simulink model "validation_simulations"  (R2019b)
settings: Solver=FixedStepAuto  StartTime=0.0  StopTime=stopTime  FixedStep=0.002  RelTol=1e-3
values from neighbouring files (symbols this model uses):
  Ao = A-L*C    [StabilizationControl.m]
  Bo = [B,L]    [StabilizationControl.m]
  Co = eye(4)    [StabilizationControl.m]
  Klqi_int = Klqi(5)    [StabilizationControl.m]
  Klqi_state = Klqi(1:4)    [StabilizationControl.m]
  Kpp_int = Kpp_i(5)    [StabilizationControl.m]
  Kpp_state = Kpp_i(1:4)    [StabilizationControl.m]
undefined symbols (not defined in the file or in its folder): ampl, ContrMethod, frequency, kalmf, Parameters
settings Model: Creator=Samsung  LastModifiedBy=Galbanyno

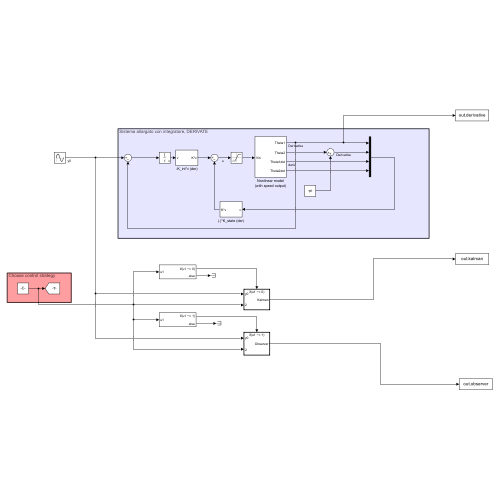
[thumbnail: Simulink's stored preview of the top-level diagram]
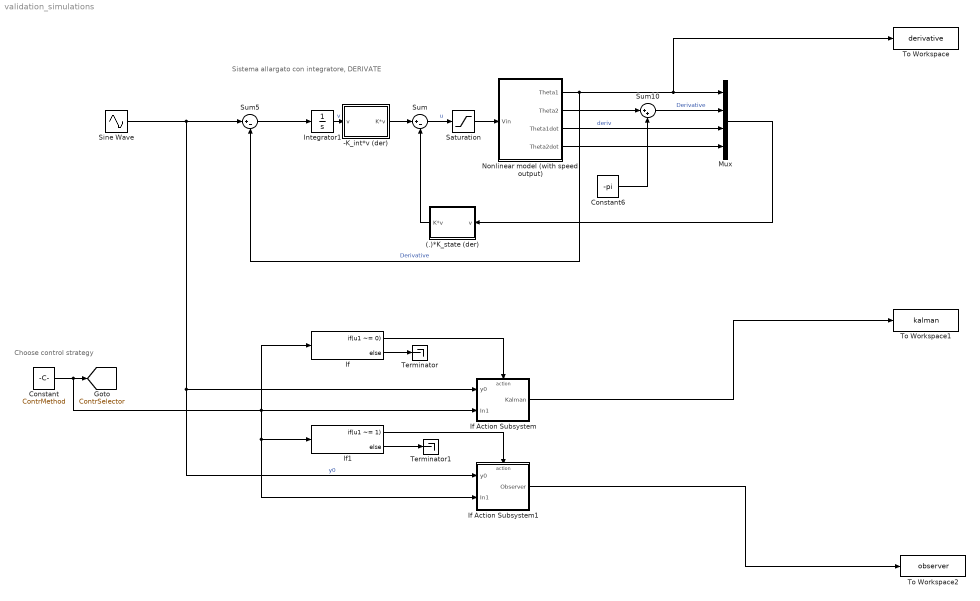
== system validation_simulations ==
  note: Choose control strategy
  note: Sistema allargato con integratore, DERIVATE
  "(.)*K_state (der) " : Subsystem
  -K_int*v (der) : Subsystem
  Constant : Constant  Value=ContrMethod
  Constant6 : Constant  Value=-pi
  If : If  IfExpression=u1 ~= 0
  If Action Subsystem : Subsystem  TreatAsAtomicUnit=on
  If Action Subsystem1 : Subsystem  TreatAsAtomicUnit=on
  If1 : If  IfExpression=u1 ~= 1
  Integrator1 : Integrator
  Mux : Mux
  Nonlinear model (with speed output) : Subsystem
  Saturation : Saturate  UpperLimit=10  LowerLimit=-10
  Sine Wave : Sin  Amplitude=ampl  Frequency=frequency  SampleTime=0
  Sum : Sum  Inputs=|+-
  Sum10 : Sum  Inputs=|++
  Sum5 : Sum  Inputs=|+-
  Terminator : Terminator
  Terminator1 : Terminator
  To Workspace : ToWorkspace  VariableName=derivative  SampleTime=-1
  To Workspace1 : ToWorkspace  VariableName=kalman  SampleTime=-1
  To Workspace2 : ToWorkspace  VariableName=observer  SampleTime=-1
  tag scope: ContrSelector=global
  wires:
  Nonlinear model (with speed output)/2(Theta2) -> Sum10/1
  "(.)*K_state (der) "/1(K*v) -> Sum/2
  Sum/1 -> Saturation/1  "u"
  Constant6/1 -> Sum10/2
  Integrator1/1 -> -K_int*v (der)/1(v)  "v"
  -K_int*v (der)/1(K*v) -> Sum/1
  Saturation/1 -> Nonlinear model (with speed output)/1(Vin)
  Sine Wave/1 -> If Action Subsystem1/1(y0), If Action Subsystem/1(y0), Sum5/1  "y0"
  Constant/1 -> If Action Subsystem/2(In1), If Action Subsystem1/2(In1), If1/1, If/1, [ContrSelector]
  Nonlinear model (with speed output)/1(Theta1) -> To Workspace/1, Mux/1, Sum5/2  "Derivative"
  Sum10/1 -> Mux/2  "Derivative"
  Nonlinear model (with speed output)/3(Theta1dot) -> Mux/3  "deriv"
  Nonlinear model (with speed output)/4(Theta2dot) -> Mux/4
  Mux/1 -> "(.)*K_state (der) "/1(v)
  Sum5/1 -> Integrator1/1
  If Action Subsystem/1(Kalman) -> To Workspace1/1
  If/1 -> If Action Subsystem/Action
  If Action Subsystem1/1(Observer) -> To Workspace2/1
  If/2 -> Terminator/1
  If1/2 -> Terminator1/1
  If1/1 -> If Action Subsystem1/Action

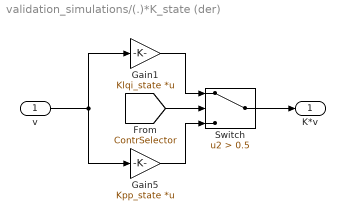
== system validation_simulations/(.)*K_state (der)  ==
  v : Inport
  Gain1 : Gain  Gain=Klqi_state  Multiplication=Matrix(K*u)
  Gain5 : Gain  Gain=Kpp_state  Multiplication=Matrix(K*u)
  Switch : Switch  Criteria=u2 > Threshold  Threshold=0.5
  K*v : Outport
  wires:
  Switch/1 -> K*v/1
  Gain5/1 -> Switch/3
  Gain1/1 -> Switch/1
  v/1 -> Gain5/1, Gain1/1
  [ContrSelector] -> Switch/2

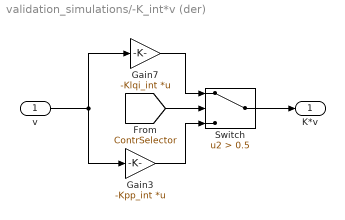
== system validation_simulations/-K_int*v (der) ==
  v : Inport
  Gain3 : Gain  Gain=-Kpp_int  Multiplication=Matrix(K*u)
  Gain7 : Gain  Gain=-Klqi_int  Multiplication=Matrix(K*u)
  Switch : Switch  Criteria=u2 > Threshold  Threshold=0.5
  K*v : Outport
  wires:
  Switch/1 -> K*v/1
  Gain3/1 -> Switch/3
  Gain7/1 -> Switch/1
  v/1 -> Gain3/1, Gain7/1
  [ContrSelector] -> Switch/2

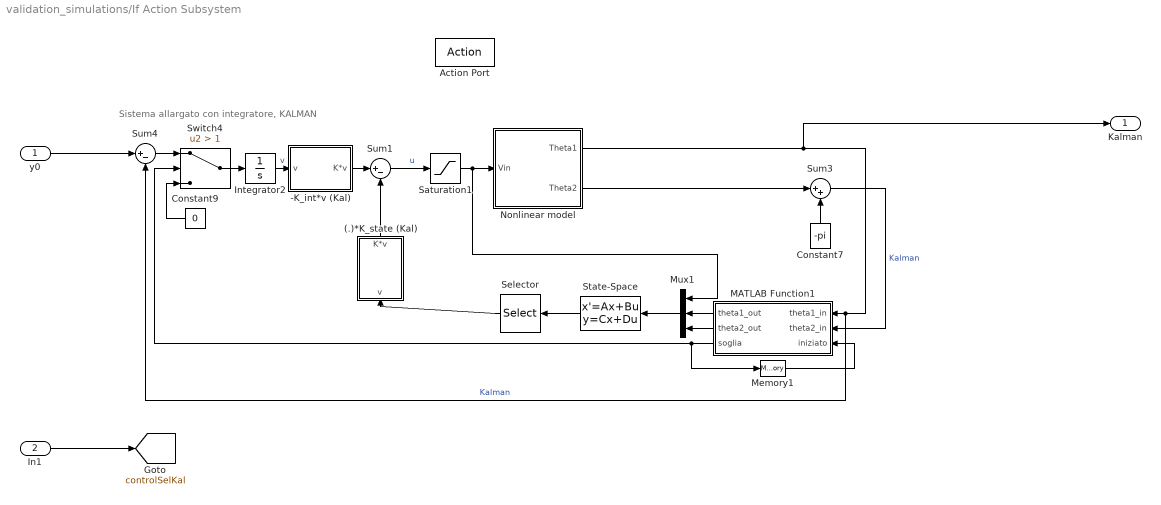
== system validation_simulations/If Action Subsystem ==
  note: Sistema allargato con integratore, KALMAN
  y0 : Inport
  In1 : Inport  Port=2
  Action Port : ActionPort  ActionPortLabel=if(u1 ~= 0)
  (.)*K_state (Kal) : Subsystem
  -K_int*v (Kal) : Subsystem
  Constant7 : Constant  Value=-pi
  Constant9 : Constant  Value=0
  Integrator2 : Integrator
  MATLAB Function1 : MATLAB Function  TreatAsAtomicUnit=on
  Memory1 : Memory  InitialCondition=false
  Mux1 : Mux  Inputs=3
  Nonlinear model : Subsystem
  Saturation1 : Saturate  UpperLimit=10  LowerLimit=-10
  Selector : Selector  InputPortWidth=6  IndexOptions=Index vector (dialog)  Indices=[3,4,5,6]  OutputSizes=1
  State-Space : StateSpace  A=kalmf.A  B=kalmf.B  C=kalmf.C  D=kalmf.D  InitialCondition=[0,0,0,0]
  Sum1 : Sum  Inputs=|+-
  Sum3 : Sum  Inputs=|++
  Sum4 : Sum  Inputs=|+-
  Switch4 : Switch  Criteria=u2 > Threshold  Threshold=1
  Kalman : Outport
  tag scope: controlSelKal=global
  wires:
  Selector/1 -> (.)*K_state (Kal)/1(v)
  Nonlinear model/2(Theta2) -> Sum3/1
  MATLAB Function1/2(theta2_out) -> Mux1/3
  (.)*K_state (Kal)/1(K*v) -> Sum1/2
  Integrator2/1 -> -K_int*v (Kal)/1(v)  "v"
  Sum3/1 -> MATLAB Function1/2(theta2_in)  "Kalman"
  Sum4/1 -> Switch4/1
  -K_int*v (Kal)/1(K*v) -> Sum1/1
  Switch4/1 -> Integrator2/1
  Constant9/1 -> Switch4/3
  Memory1/1 -> MATLAB Function1/3(iniziato)
  State-Space/1 -> Selector/1
  y0/1 -> Sum4/1
  Sum1/1 -> Saturation1/1  "u"
  MATLAB Function1/1(theta1_out) -> Mux1/2
  In1/1 -> [controlSelKal]
  Saturation1/1 -> Mux1/1, Nonlinear model/1(Vin)
  Nonlinear model/1(Theta1) -> Kalman/1, MATLAB Function1/1(theta1_in), Sum4/2  "Kalman"
  MATLAB Function1/3(soglia) -> Memory1/1, Switch4/2
  Mux1/1 -> State-Space/1
  Constant7/1 -> Sum3/2

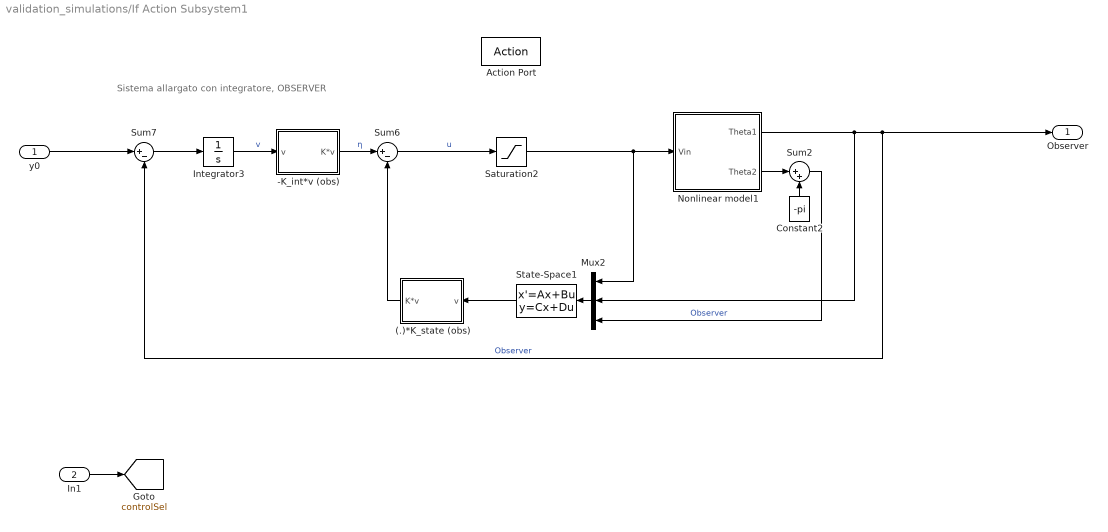
== system validation_simulations/If Action Subsystem1 ==
  note: Sistema allargato con integratore, OBSERVER
  y0 : Inport
  In1 : Inport  Port=2
  Action Port : ActionPort  ActionPortLabel=if(u1 ~= 1)
  (.)*K_state (obs) : Subsystem
  -K_int*v (obs) : Subsystem
  Constant2 : Constant  Value=-pi
  Integrator3 : Integrator
  Mux2 : Mux  Inputs=3
  Nonlinear model1 : Subsystem
  Saturation2 : Saturate  UpperLimit=10  LowerLimit=-10
  State-Space1 : StateSpace  A=Ao  B=Bo  C=Co  D=zeros(4,3)  InitialCondition=[0,0,0,0]
  Sum2 : Sum  Inputs=|++
  Sum6 : Sum  Inputs=|+-
  Sum7 : Sum  Inputs=|+-
  Observer : Outport
  tag scope: controlSel=global
  wires:
  In1/1 -> [controlSel]
  Nonlinear model1/2(Theta2) -> Sum2/1
  Sum2/1 -> Mux2/3  "Observer"
  Sum7/1 -> Integrator3/1
  -K_int*v (obs)/1(K*v) -> Sum6/1  "η"
  (.)*K_state (obs)/1(K*v) -> Sum6/2
  Sum6/1 -> Saturation2/1  "u"
  y0/1 -> Sum7/1
  Constant2/1 -> Sum2/2
  Saturation2/1 -> Mux2/1, Nonlinear model1/1(Vin)
  State-Space1/1 -> (.)*K_state (obs)/1(v)
  Nonlinear model1/1(Theta1) -> Mux2/2, Observer/1, Sum7/2  "Observer"
  Mux2/1 -> State-Space1/1
  Integrator3/1 -> -K_int*v (obs)/1(v)  "v"

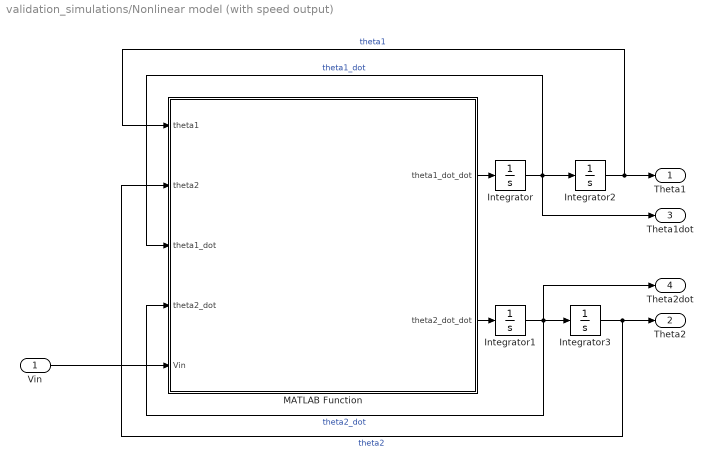
== system validation_simulations/Nonlinear model (with speed output) ==
  Vin : Inport
  Integrator : Integrator  InitialCondition=0.05
  Integrator1 : Integrator  InitialCondition=0.05
  Integrator2 : Integrator
  Integrator3 : Integrator  InitialCondition=pi
  MATLAB Function : MATLAB Function  TreatAsAtomicUnit=on  mask{Pars=Parameters}
      mask prompts: Pars "Struct containing model parameters"
  Theta1 : Outport
  Theta2 : Outport  Port=2
  Theta1dot : Outport  Port=3
  Theta2dot : Outport  Port=4
  wires:
  Integrator/1 -> Theta1dot/1, MATLAB Function/3(theta1_dot), Integrator2/1  "theta1_dot"
  Integrator1/1 -> Theta2dot/1, MATLAB Function/4(theta2_dot), Integrator3/1  "theta2_dot"
  MATLAB Function/1(theta1_dot_dot) -> Integrator/1
  Integrator3/1 -> Theta2/1, MATLAB Function/2(theta2)  "theta2"
  MATLAB Function/2(theta2_dot_dot) -> Integrator1/1
  Integrator2/1 -> MATLAB Function/1(theta1), Theta1/1  "theta1"
  Vin/1 -> MATLAB Function/5(Vin)

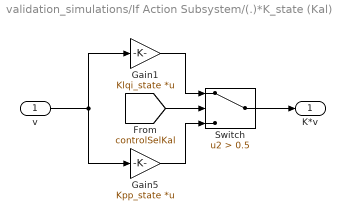
== system validation_simulations/If Action Subsystem/(.)*K_state (Kal) ==
  v : Inport
  Gain1 : Gain  Gain=Klqi_state  Multiplication=Matrix(K*u)
  Gain5 : Gain  Gain=Kpp_state  Multiplication=Matrix(K*u)
  Switch : Switch  Criteria=u2 > Threshold  Threshold=0.5
  K*v : Outport
  wires:
  Switch/1 -> K*v/1
  Gain5/1 -> Switch/3
  Gain1/1 -> Switch/1
  v/1 -> Gain5/1, Gain1/1
  [controlSelKal] -> Switch/2

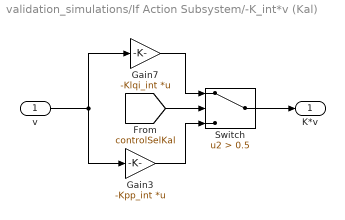
== system validation_simulations/If Action Subsystem/-K_int*v (Kal) ==
  v : Inport
  Gain3 : Gain  Gain=-Kpp_int  Multiplication=Matrix(K*u)
  Gain7 : Gain  Gain=-Klqi_int  Multiplication=Matrix(K*u)
  Switch : Switch  Criteria=u2 > Threshold  Threshold=0.5
  K*v : Outport
  wires:
  Switch/1 -> K*v/1
  Gain3/1 -> Switch/3
  Gain7/1 -> Switch/1
  v/1 -> Gain3/1, Gain7/1
  [controlSelKal] -> Switch/2

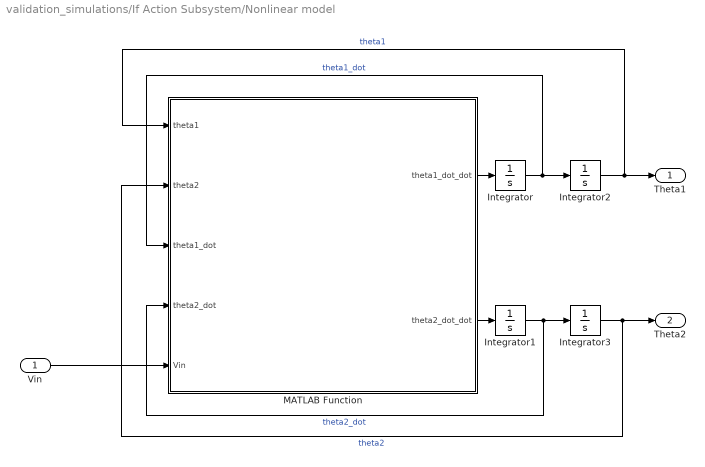
== system validation_simulations/If Action Subsystem/Nonlinear model ==
  Vin : Inport
  Integrator : Integrator  InitialCondition=0.05
  Integrator1 : Integrator  InitialCondition=0.05
  Integrator2 : Integrator
  Integrator3 : Integrator  InitialCondition=pi
  MATLAB Function : MATLAB Function  TreatAsAtomicUnit=on  mask{Pars=Parameters}
      mask prompts: Pars "Struct containing model parameters"
  Theta1 : Outport
  Theta2 : Outport  Port=2
  wires:
  Integrator/1 -> MATLAB Function/3(theta1_dot), Integrator2/1  "theta1_dot"
  Integrator1/1 -> MATLAB Function/4(theta2_dot), Integrator3/1  "theta2_dot"
  MATLAB Function/1(theta1_dot_dot) -> Integrator/1
  Integrator3/1 -> Theta2/1, MATLAB Function/2(theta2)  "theta2"
  MATLAB Function/2(theta2_dot_dot) -> Integrator1/1
  Integrator2/1 -> MATLAB Function/1(theta1), Theta1/1  "theta1"
  Vin/1 -> MATLAB Function/5(Vin)

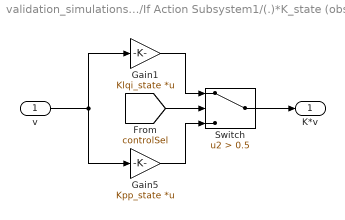
== system validation_simulations/If Action Subsystem1/(.)*K_state (obs) ==
  v : Inport
  Gain1 : Gain  Gain=Klqi_state  Multiplication=Matrix(K*u)
  Gain5 : Gain  Gain=Kpp_state  Multiplication=Matrix(K*u)
  Switch : Switch  Criteria=u2 > Threshold  Threshold=0.5
  K*v : Outport
  wires:
  Switch/1 -> K*v/1
  Gain5/1 -> Switch/3
  Gain1/1 -> Switch/1
  v/1 -> Gain5/1, Gain1/1
  [controlSel] -> Switch/2

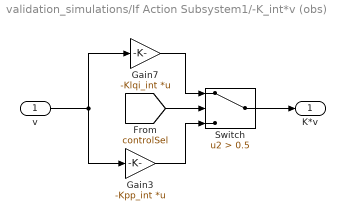
== system validation_simulations/If Action Subsystem1/-K_int*v (obs) ==
  v : Inport
  Gain3 : Gain  Gain=-Kpp_int  Multiplication=Matrix(K*u)
  Gain7 : Gain  Gain=-Klqi_int  Multiplication=Matrix(K*u)
  Switch : Switch  Criteria=u2 > Threshold  Threshold=0.5
  K*v : Outport
  wires:
  Switch/1 -> K*v/1
  Gain3/1 -> Switch/3
  Gain7/1 -> Switch/1
  v/1 -> Gain3/1, Gain7/1
  [controlSel] -> Switch/2

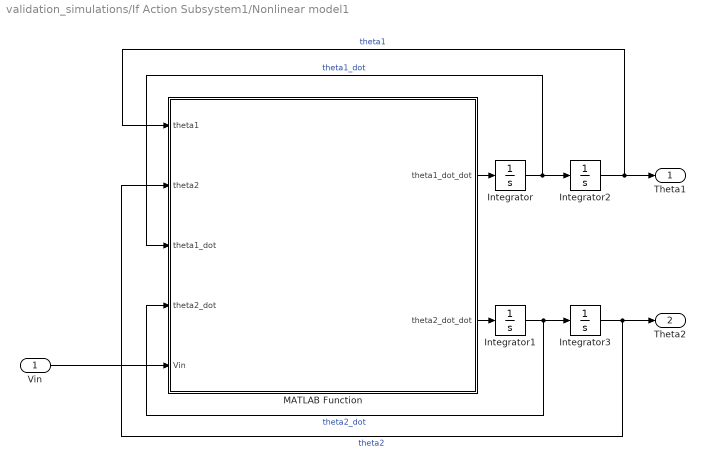
== system validation_simulations/If Action Subsystem1/Nonlinear model1 ==
  Vin : Inport
  Integrator : Integrator  InitialCondition=0.05
  Integrator1 : Integrator  InitialCondition=0.05
  Integrator2 : Integrator
  Integrator3 : Integrator  InitialCondition=pi
  MATLAB Function : MATLAB Function  TreatAsAtomicUnit=on  mask{Pars=Parameters}
      mask prompts: Pars "Struct containing model parameters"
  Theta1 : Outport
  Theta2 : Outport  Port=2
  wires:
  Integrator/1 -> MATLAB Function/3(theta1_dot), Integrator2/1  "theta1_dot"
  Integrator1/1 -> MATLAB Function/4(theta2_dot), Integrator3/1  "theta2_dot"
  MATLAB Function/1(theta1_dot_dot) -> Integrator/1
  Integrator3/1 -> Theta2/1, MATLAB Function/2(theta2)  "theta2"
  MATLAB Function/2(theta2_dot_dot) -> Integrator1/1
  Integrator2/1 -> MATLAB Function/1(theta1), Theta1/1  "theta1"
  Vin/1 -> MATLAB Function/5(Vin)

== matlab function validation_simulations/Nonlinear model (with speed output)/MATLAB Function ==
  data: theta1 input; theta1_dot_dot output; theta2 input; theta1_dot input; theta2_dot input; Vin input; theta2_dot_dot output; Pars parameter
function [theta1_dot_dot,theta2_dot_dot] = fcn(theta1, theta2, theta1_dot, theta2_dot,Vin, Pars)

   k1 = Pars.Jeq + Pars.m2*(Pars.l1^2 + Pars.x2^2*sin(theta2)^2);
   k2 = Pars.m2*Pars.l1*Pars.x2*cos(theta2);
   k3 = 2*Pars.m2*Pars.x2^2*sin(theta2)*cos(theta2)*theta1_dot*theta2_dot - Pars.m2*Pars.l1*Pars.x2*sin(theta2)*theta2_dot^2 +Pars.Ks*theta1 - Pars.Km/Pars.Rm*Vin + (Pars.Km^2)/Pars.Rm*theta1_dot + Pars.Kf1*theta1_dot;
   k4 = Pars.m2*Pars.l1*Pars.x2*cos(theta2);
   k5 = Pars.m2*Pars.x2^2 + Pars.I2;
   k6 = - Pars.m2*Pars.x2^2*sin(theta2)*cos(theta2)*theta1_dot^2 + Pars.m2*Pars.g*Pars.x2*sin(theta2) + Pars.Kf2*theta2_dot;


theta1_dot_dot = (k2*k6 - k3*k5)/(k1*k5 - k2*k4);
theta2_dot_dot = -(k1*k6 - k3*k4)/(k1*k5 - k2*k4);

== matlab function validation_simulations/If Action Subsystem1/Nonlinear model1/MATLAB Function ==
  data: theta1 input; theta1_dot_dot output; theta2 input; theta1_dot input; theta2_dot input; Vin input; theta2_dot_dot output; Pars parameter
function [theta1_dot_dot,theta2_dot_dot] = fcn(theta1, theta2, theta1_dot, theta2_dot,Vin, Pars)

   k1 = Pars.Jeq + Pars.m2*(Pars.l1^2 + Pars.x2^2*sin(theta2)^2);
   k2 = Pars.m2*Pars.l1*Pars.x2*cos(theta2);
   k3 = 2*Pars.m2*Pars.x2^2*sin(theta2)*cos(theta2)*theta1_dot*theta2_dot - Pars.m2*Pars.l1*Pars.x2*sin(theta2)*theta2_dot^2 +Pars.Ks*theta1 - Pars.Km/Pars.Rm*Vin + (Pars.Km^2)/Pars.Rm*theta1_dot + Pars.Kf1*theta1_dot;
   k4 = Pars.m2*Pars.l1*Pars.x2*cos(theta2);
   k5 = Pars.m2*Pars.x2^2 + Pars.I2;
   k6 = - Pars.m2*Pars.x2^2*sin(theta2)*cos(theta2)*theta1_dot^2 + Pars.m2*Pars.g*Pars.x2*sin(theta2) + Pars.Kf2*theta2_dot;


theta1_dot_dot = (k2*k6 - k3*k5)/(k1*k5 - k2*k4);
theta2_dot_dot = -(k1*k6 - k3*k4)/(k1*k5 - k2*k4);

== matlab function validation_simulations/If Action Subsystem/MATLAB Function1 ==
  data: theta1_in input; theta1_out output; theta2_in input; iniziato input double; theta2_out output; soglia output
function [theta1_out, theta2_out, soglia] = fcn(theta1_in, theta2_in, iniziato)
if theta2_in >= 0.01
    theta1_out = theta1_in;
    theta2_out = theta2_in;
    soglia = 2; 
elseif iniziato >1
    theta1_out = theta1_in;
    theta2_out = theta2_in;
    soglia = 2;
else
    soglia = 0;
    theta1_out = 0;
    theta2_out = 0;
end
% soglia = 2;s
% theta1_out = theta1_in;
% theta2_out = theta2_in;
end

== matlab function validation_simulations/If Action Subsystem/Nonlinear model/MATLAB Function ==
  data: theta1 input; theta1_dot_dot output; theta2 input; theta1_dot input; theta2_dot input; Vin input; theta2_dot_dot output; Pars parameter
function [theta1_dot_dot,theta2_dot_dot] = fcn(theta1, theta2, theta1_dot, theta2_dot,Vin, Pars)

   k1 = Pars.Jeq + Pars.m2*(Pars.l1^2 + Pars.x2^2*sin(theta2)^2);
   k2 = Pars.m2*Pars.l1*Pars.x2*cos(theta2);
   k3 = 2*Pars.m2*Pars.x2^2*sin(theta2)*cos(theta2)*theta1_dot*theta2_dot - Pars.m2*Pars.l1*Pars.x2*sin(theta2)*theta2_dot^2 +Pars.Ks*theta1 - Pars.Km/Pars.Rm*Vin + (Pars.Km^2)/Pars.Rm*theta1_dot + Pars.Kf1*theta1_dot;
   k4 = Pars.m2*Pars.l1*Pars.x2*cos(theta2);
   k5 = Pars.m2*Pars.x2^2 + Pars.I2;
   k6 = - Pars.m2*Pars.x2^2*sin(theta2)*cos(theta2)*theta1_dot^2 + Pars.m2*Pars.g*Pars.x2*sin(theta2) + Pars.Kf2*theta2_dot;


theta1_dot_dot = (k2*k6 - k3*k5)/(k1*k5 - k2*k4);
theta2_dot_dot = -(k1*k6 - k3*k4)/(k1*k5 - k2*k4);
